simulink model "prob3"  (R2020a)
settings: Solver=VariableStepAuto  StartTime=0.0  StopTime=120  RelTol=1e-3
values from neighbouring files (symbols this model uses):
  b = 50.0    [dict.sldd]
  ki = 40.0    [dict.sldd]
  kp = 800.0    [dict.sldd]
  m = 1000.0    [dict.sldd]
settings Model: DataDictionary=dict.sldd  Creator=I3  LastModifiedBy=I3

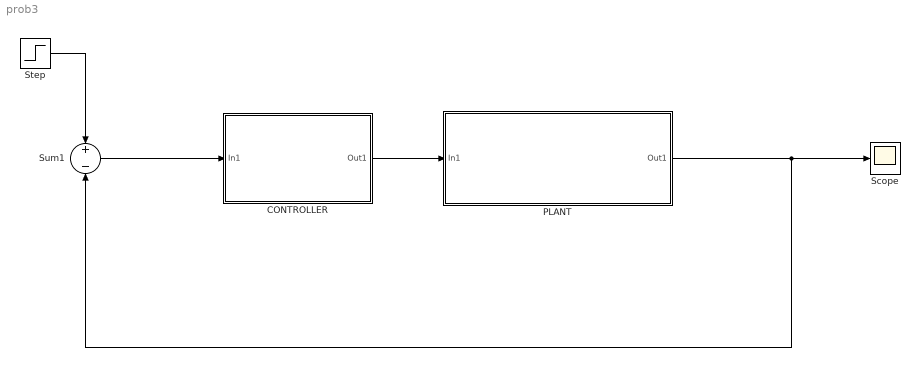
== system prob3 ==
  CONTROLLER : Subsystem
  PLANT : Subsystem
  Scope : Scope
  Step : Step  After=u  SampleTime=0
  Sum1 : Sum  Inputs=+-
  wires:
  PLANT/1(Out1) -> Sum1/2, Scope/1
  Step/1 -> Sum1/1
  Sum1/1 -> CONTROLLER/1(In1)
  CONTROLLER/1(Out1) -> PLANT/1(In1)

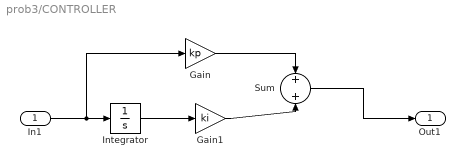
== system prob3/CONTROLLER ==
  In1 : Inport
  Gain : Gain  Gain=kp
  Gain1 : Gain  Gain=ki
  Integrator : Integrator
  Sum : Sum
  Out1 : Outport
  wires:
  Sum/1 -> Out1/1
  In1/1 -> Gain/1, Integrator/1
  Integrator/1 -> Gain1/1
  Gain1/1 -> Sum/2
  Gain/1 -> Sum/1

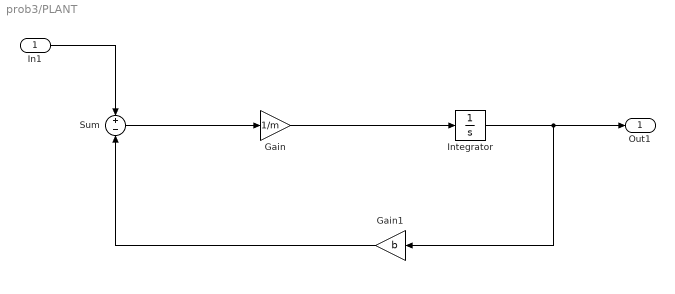
== system prob3/PLANT ==
  In1 : Inport
  Gain : Gain  Gain=1/m
  Gain1 : Gain  Gain=b
  Integrator : Integrator
  Sum : Sum  Inputs=+-
  Out1 : Outport
  wires:
  Gain1/1 -> Sum/2
  Integrator/1 -> Out1/1, Gain1/1
  Sum/1 -> Gain/1
  Gain/1 -> Integrator/1
  In1/1 -> Sum/1
